simulink model "afe_abc_inv_psm_n"  (R2025b)
settings: Solver=ode1  StartTime=0.0  StopTime=simlength  FixedStep=tc  MaxStep=tc
values from neighbouring files (symbols this model uses):
  Adrso = eye(2) + Arso*ts_afe    [init_model.m]
  afe_pwm_phase_shift_mod1 = 0    [init_model.m]
  afe_pwm_phase_shift_mod2 = 0    [init_model.m]
  Aresd = eye(2) + Ares*ts_afe    [init_model.m]
  Bresd = Bres*ts_afe    [init_model.m]
  Cresd = Cres    [init_model.m]
  Crso = [1 0]    [init_model.m]
  CTRPIFF_CLIP_RELEASE = 0.001    [init_model.m]
  deepNEGeta = 0.5    [init_model.m]
  deepNEGxi = 0    [init_model.m]
  deepPOSxi = 0.5    [init_model.m]
  emf_fb_p = 0.2    [init_model.m]
  emf_fb_p_ccaller_1 = emf_fb_p    (= 0.2)    [init_model.m]
  emf_fb_p_ccaller_2 = emf_fb_p    (= 0.2)    [init_model.m]
  emf_p = emf_fb_p*4/10    (= 0.08)    [init_model.m]
  emf_p_ccaller_1 = emf_fb_p_ccaller_1*4/10    (= 0.08)    [init_model.m]
  emf_p_ccaller_2 = emf_fb_p_ccaller_2*4/10    (= 0.08)    [init_model.m]
  g0_161Hz = fcut_161Hz_flt * ts_afe * 2*pi    (= 0.126449104307)    [init_model.m]
  g0_1Hz = fcut_1Hz_flt * ts_afe * 2*pi    (= 0.000785398163397)    [init_model.m]
  g0_500Hz = fcut_500Hz_flt * ts_afe * 2*pi    (= 0.392699081699)    [init_model.m]
  g1_161Hz = 1 - g0_161Hz    (= 0.873550895693)    [init_model.m]
  g1_1Hz = 1 - g0_1Hz    (= 0.999214601837)    [init_model.m]
  g1_500Hz = 1 - g0_500Hz    (= 0.607300918301)    [init_model.m]
  i_grid_neg_eta_lim = 0.5    [init_model.m]
  i_grid_neg_eta_red_lim = 0.1    [init_model.m]
  i_grid_neg_xi_lim = 0.5    [init_model.m]
  i_grid_neg_xi_red_lim = 0.1    [init_model.m]
  i_grid_pos_eta_lim = 1    [init_model.m]
  i_grid_pos_eta_red_lim = 0.1    [init_model.m]
  id_lim = 0.35    [init_model.m]
  ieta_neg_ref_lim = 0.5    [init_model.m]
  ieta_pos_ref_lim = 1.0    (= 1)    [init_model.m]
  Igrid_phase_normalization_factor = 250e3/Vphase2/3/0.9*sqrt(2)    [init_model.m]
  inv_pwm_phase_shift_mod1 = 0    [init_model.m]
  iq_lim = 1.4    [init_model.m]
  ixi_pos_ref_lim = 1.6    [init_model.m]
  k_frt_ref = 2    [init_model.m]
  kg = Kobs(1)    [init_model.m]
  ki_afe = 45    [init_model.m]
  ki_align = 0.1    [init_model.m]
  ki_i = 18    [init_model.m]
  ki_rc_neg_grid = ki_rc_grid    (= 35)    [init_model.m]
  ki_rc_pos_grid = ki_rc_grid    (= 35)    [init_model.m]
  ki_vs = 35    [init_model.m]
  ki_w = 18    [init_model.m]
  kp_afe = 0.6    [init_model.m]
  kp_align = 0.6    [init_model.m]
  kp_i = 0.25    [init_model.m]
  kp_rc_neg_grid = kp_rc_grid    (= 0.35)    [init_model.m]
  kp_rc_pos_grid = kp_rc_grid    (= 0.35)    [init_model.m]
  kp_vs = 0.85    [init_model.m]
  kp_w = 2.5    [init_model.m]
  kw = Kobs(2)    [init_model.m]
  l1 = Kd(2)    [init_model.m]
  l2 = Kd(1)    [init_model.m]
  Ldrso = acker(Adrso',Crso',polesdrso)'    [init_model.m]
  lim_down_align = -0.2    [init_model.m]
  lim_up_align = 0.2    [init_model.m]
  mavarage_filter_frequency_base_order = 2    [init_model.m]
  motorc_m_scale = 2/3*Vdc_bez/ubez    [init_model.m]
  n1 = rms_perios/f_grid/ts_afe    [init_model.m]
  n10 = rms_perios/f_grid/ts_afe    [init_model.m]
  number_of_modules = 2    [init_model.m]
  omega_m_sim = omega_m_bez    [init_model.m]
  pll_i1 = 80    [init_model.m]
  pll_i1_ddsrt = pll_i1/2    (= 40)    [init_model.m]
  pll_p = 1    [init_model.m]
  pll_p_ddsrt = pll_p/2    (= 0.5)    [init_model.m]
  pll_p_frt = 0.2    [init_model.m]
  settle_time = 0.15    [init_model.m]
  simlength = 2    [init_model.m]
  start_time_LVRT = 2.0    (= 2)    [init_model.m]
  tc = ts_afe/200    (= 6.25e-07)    [init_model.m]
  time_aux_power_supply_fault = 1e3    (= 1000)    [init_model.m]
  time_gain_afe_module_1 = 1.0    (= 1)    [init_model.m]
  time_gain_afe_module_2 = 1.0    (= 1)    [init_model.m]
  time_gain_inv_module_1 = 1.0    (= 1)    [init_model.m]
  time_gain_inv_module_2 = 1.0    (= 1)    [init_model.m]
  time_phase_fault = 1e3    (= 1000)    [init_model.m]
  time_start_motor_control = 0.035    [init_model.m]
  transmission_delay = 125e-6*2    (= 0.00025)    [init_model.m]
  ts_afe = 1/fPWM_AFE/2    (= 0.000125)    [init_model.m]
  ts_inv = 1/fPWM_INV/2    (= 0.000125)    [init_model.m]
  Vdc_norm_ref = Vdc_ref/Vdc_nom    [init_model.m]
  Vdc_ref = 1070    [init_model.m]
  Vgrid_phase_normalization_factor = Vphase2*sqrt(2)    [init_model.m]
undefined symbols (not defined in the file or in its folder): Amplitude_U, Amplitude_V, Amplitude_W, end_time_LVRT, ibez, La, Lb, Ld_norm, Lq_norm, Ls_norm, magnitude, omega_bez, omega_grid_emulator_nom, omega_grid_nom, omega_m_bez, Phase_shift, psi_bez, psi_m, psi_m_norm, rpm_base, rpm_bez, Rs, Rs_norm, t_ramp, tau_bez, torque_base, ubez, ugrid_factor, V_phase_normalization_factor, Vdc_bez, Vemu_ref_norm, vn_eta_pu, vn_xi_pu, vp_xi_pu
libraries: fl_lib x215, nesl_utility x107, moving_average_filter x20, cstblocks x20, moving_average_filter_cc x16, simulink x6, threephase_inductor_lib x4, three_phase_pwm_modulator x4, single_phase_transformer_lib x3, power_meter_iec x1, flexshaft_lib x1, psm x1
(part 6 of 15)

== system afe_abc_inv_psm_n/afe_abc_inv_psm_mod1/AFE_control/afe_control/udc_ctrl ==
  udc_pu : Inport
  udc_pu_ref : Inport  Port=2
  1/Ti : Gain  Gain=kp_vs  SaturateOnIntegerOverflow=on  OutDataTypeStr=Inherit: Same as input  ParamDataTypeStr=Inherit: Same as input
  Constant : Constant  Value=0
  Gain : Gain  Gain=-1
  Saturation : Saturate  UpperLimit=ixi_pos_ref_lim  LowerLimit=-ixi_pos_ref_lim
  Sum1 : Sum  Inputs=+++  SaturateOnIntegerOverflow=on
  Sum2 : Sum  Inputs=-+  SaturateOnIntegerOverflow=on
  Sum3 : Sum  Inputs=-+  SaturateOnIntegerOverflow=on
  Switch : Switch  Criteria=u2 > Threshold  SaturateOnIntegerOverflow=off  InputSameDT=off
  To Workspace1 : ToWorkspace  VariableName=udc_pu_sim_mod1  SampleTime=-1
      settings: MaxDataPoints=Ns_afe
  To Workspace3 : ToWorkspace  VariableName=udc_pu_ref_sim_mod1  SampleTime=-1
      settings: MaxDataPoints=Ns_afe
  Unit Delay4 : UnitDelay  SampleTime=-1  HasFrameUpgradeWarning=on
  kp : Gain  Gain=ki_vs*ts_afe  SaturateOnIntegerOverflow=on  OutDataTypeStr=Inherit: Same as input  ParamDataTypeStr=Inherit: Same as input
  udc_tracking : Scope  NumInputPorts=2
      settings: ActiveDisplayYMinimum=-0.14752197265624997  ActiveDisplayYMaximum=1.32769775390625  DataLoggingVariableName=ScopeData8
  i_xi_ref : Outport
  wires:
  1/Ti/1 -> Sum1/1, Sum3/1
  kp/1 -> Sum1/2
  Sum3/1 -> Unit Delay4/1
  Unit Delay4/1 -> Sum1/3
  udc_pu_ref/1 -> To Workspace3/1, udc_tracking/1, Sum2/2  "udc_pu_ref"
  udc_pu/1 -> To Workspace1/1, udc_tracking/2, Sum2/1  "udc_pu"
  Sum2/1 -> kp/1, 1/Ti/1
  Sum1/1 -> Saturation/1
  Saturation/1 -> Gain/1, Sum3/2
  [pwr_lim_enable_mod1] -> Switch/2
  Gain/1 -> Switch/3
  Switch/1 -> i_xi_ref/1
  Constant/1 -> Switch/1

== system afe_abc_inv_psm_n/afe_abc_inv_psm_mod1/AFE_control/afe_control/ug afe quantizzation and one step delay ==
  ug_abc_pu : Inport
  Demux : Demux  Outputs=3
  Mux : Mux  Inputs=3
  ug afe quantizzation and one step delay : Subsystem
  ugd_abc_pu : Outport
  wires:
  ug afe quantizzation and one step delay/2(ugd_v_pu) -> Mux/2
  Demux/2 -> ug afe quantizzation and one step delay/2(ug_v_pu)
  Demux/3 -> ug afe quantizzation and one step delay/3(ug_w_pu)
  ug afe quantizzation and one step delay/1(ugd_u_pu) -> Mux/1
  Demux/1 -> ug afe quantizzation and one step delay/1(ug_u_pu)
  ug_abc_pu/1 -> Demux/1
  ug afe quantizzation and one step delay/3(ugd_w_pu) -> Mux/3
  Mux/1 -> ugd_abc_pu/1

== system afe_abc_inv_psm_n/afe_abc_inv_psm_mod1/INV_control/inverter_control/Speed control ==
  rotor speed : Inport
  rotor speed ref : Inport  Port=2
  1/Ti : Gain  Gain=kp_w  SaturateOnIntegerOverflow=on  OutDataTypeStr=Inherit: Same as input  ParamDataTypeStr=Inherit: Same as input
  Saturation : Saturate  UpperLimit=iq_lim  LowerLimit=-iq_lim
  Sum1 : Sum  Inputs=+++  SaturateOnIntegerOverflow=on
  Sum2 : Sum  Inputs=-+  SaturateOnIntegerOverflow=on
  Sum3 : Sum  Inputs=-+  SaturateOnIntegerOverflow=on
  Unit Delay4 : UnitDelay  SampleTime=-1  HasFrameUpgradeWarning=on
  kp : Gain  Gain=ki_w*ts_inv  SaturateOnIntegerOverflow=on  OutDataTypeStr=Inherit: Same as input  ParamDataTypeStr=Inherit: Same as input
  torque_ref : Outport
  wires:
  1/Ti/1 -> Sum1/1, Sum3/1
  kp/1 -> Sum1/2
  Sum3/1 -> Unit Delay4/1
  Unit Delay4/1 -> Sum1/3
  rotor speed ref/1 -> Sum2/2
  rotor speed/1 -> Sum2/1
  Sum2/1 -> kp/1, 1/Ti/1
  Sum1/1 -> Saturation/1
  Saturation/1 -> Sum3/2, torque_ref/1

== system afe_abc_inv_psm_n/afe_abc_inv_psm_mod1/INV_control/inverter_control/current_ctrl ==
  torque_ref : Inport
  Bus Creator1 : BusCreator  Inputs=2
  bemf_observer : Subsystem
  current_ctrl : Subsystem
  current_transformation : Subsystem
  uab : Outport  VectorParamsAs1DForOutWhenUnconnected=off
  wires:
  [ubeta_pu_mod1] -> Bus Creator1/2  "ub"
  [ualpha_pu_mod1] -> Bus Creator1/1  "ua"
  Bus Creator1/1 -> uab/1
  torque_ref/1 -> current_ctrl/1(iq_ref)  "torque_ref"
  [ibeta_pu_mod1] -> bemf_observer/2(ibeta_pu)
  [ialpha_pu_mod1] -> bemf_observer/1(ialpha_pu)
  [ualpha_pu_mod1] -> bemf_observer/3(ualpha_pu)
  [ubeta_pu_mod1] -> bemf_observer/4(ubeta_pu)
  [udcd_pu_inv_mod1] -> current_ctrl/2(udc_pu), bemf_observer/5(udc_pu)

== system afe_abc_inv_psm_n/afe_abc_inv_psm_mod1/INV_control/inverter_control/encoder-sensorless-switch ==
  theta_elec_psm : Inport
  Variant Source1 : VariantSource  VariantControls={use_psm_encoder == 1, use_psm_encoder == 0}
  Variant Source2 : VariantSource  VariantControls={use_psm_encoder == 1, use_psm_encoder == 0}
  double_integrator_observer : Subsystem
  omega_pu_psm/hat1 : Scope  NumInputPorts=2
      settings: ActiveDisplayYMinimum=-0.11085278602064572  ActiveDisplayYMaximum=0.99767500251710517  DataLoggingVariableName=ScopeData13
  theta_elec_psm/hat : Scope  NumInputPorts=2
      settings: ActiveDisplayYMinimum=-3.9234912991523743  ActiveDisplayYMaximum=3.9263074994087219  DataLoggingVariableName=ScopeData12
  tag scope: motor_phase_ctrl_mod1=global, motor_speed_pu_ctrl_mod1=global
  wires:
  double_integrator_observer/1(omega_pu_psm_hat) -> omega_pu_psm/hat1/2, Variant Source1/1  "omega_pu_psm_hat"
  [theta_hat_mod1] -> Variant Source2/2  "theta_hat_mod1"
  theta_elec_psm/1 -> theta_elec_psm/hat/2, double_integrator_observer/1(theta_psm)  "theta_elec_psm"
  double_integrator_observer/2(theta_psm_hat) -> Variant Source2/1  "theta_psm_hat"
  [omega_hat_pu_mod1] -> Variant Source1/2  "omega_hat_pu_mod1"
  Variant Source1/1 -> [motor_speed_pu_ctrl_mod1]
  Variant Source2/1 -> [motor_phase_ctrl_mod1]
  [theta_hat_mod1] -> theta_elec_psm/hat/1  "theta_hat_mod1"
  [omega_hat_pu_mod1] -> omega_pu_psm/hat1/1  "omega_hat_pu_mod1"

== system afe_abc_inv_psm_n/afe_abc_inv_psm_mod1/INV_control/inverter_control/is inv quantizzation and one step delay ==
  is_abc_pu : Inport
  Demux : Demux  Outputs=3
  Mux : Mux  Inputs=3
  is inv quantizzation and one step delay : Subsystem
  isd_abc_pu : Outport
  wires:
  is inv quantizzation and one step delay/2(isd_v_pu) -> Mux/2
  is_abc_pu/1 -> Demux/1
  is inv quantizzation and one step delay/3(isd_w_pu) -> Mux/3
  is inv quantizzation and one step delay/1(isd_u_pu) -> Mux/1
  Demux/1 -> is inv quantizzation and one step delay/1(is_u_pu)
  Mux/1 -> isd_abc_pu/1
  Demux/3 -> is inv quantizzation and one step delay/3(is_w_pu)
  Demux/2 -> is inv quantizzation and one step delay/2(is_v_pu)

== system afe_abc_inv_psm_n/afe_abc_inv_psm_mod1/INV_control/inverter_control/measurements ==
  Gain : Gain  Gain=psi_bez
  Gain1 : Gain  Gain=psi_bez
  To Workspace10 : ToWorkspace  VariableName=id_pu_sim_mod1  SampleTime=-1
      settings: MaxDataPoints=Ns_inv
  To Workspace11 : ToWorkspace  VariableName=iq_pu_sim_mod1  SampleTime=-1
      settings: MaxDataPoints=Ns_inv
  To Workspace12 : ToWorkspace  VariableName=uq_pu_sim_mod1  SampleTime=-1
      settings: MaxDataPoints=Ns_inv
  To Workspace13 : ToWorkspace  VariableName=iq_pu_ref_sim_mod1  SampleTime=-1
      settings: MaxDataPoints=Ns_inv
  To Workspace14 : ToWorkspace  VariableName=id_pu_ref_sim_mod1  SampleTime=-1
      settings: MaxDataPoints=Ns_inv
  To Workspace15 : ToWorkspace  VariableName=u_mot_pu_sim_mod1  SampleTime=-1
      settings: MaxDataPoints=Ns_inv
  To Workspace2 : ToWorkspace  VariableName=ualpha_pu_sim_mod1  SampleTime=-1
      settings: MaxDataPoints=Ns_inv
  To Workspace3 : ToWorkspace  VariableName=ubeta_pu_sim_mod1  SampleTime=-1
      settings: MaxDataPoints=Ns_inv
  To Workspace4 : ToWorkspace  VariableName=psi_pu_alpha_hat_sim_mod1  SampleTime=-1
      settings: MaxDataPoints=Ns_inv
  To Workspace5 : ToWorkspace  VariableName=psi_pu_beta_hat_sim_mod1  SampleTime=-1
      settings: MaxDataPoints=Ns_inv
  To Workspace6 : ToWorkspace  VariableName=psi_r_alpha_hat_sim_mod1  SampleTime=-1
      settings: MaxDataPoints=Ns_inv
  To Workspace7 : ToWorkspace  VariableName=ud_pu_sim_mod1  SampleTime=-1
      settings: MaxDataPoints=Ns_inv
  To Workspace8 : ToWorkspace  VariableName=psi_r_beta_hat_sim_mod1  SampleTime=-1
      settings: MaxDataPoints=Ns_inv
  wires:
  [psi_r_alpha_pu_hat_mod1] -> Gain/1
  [ualpha_pu_mod1] -> To Workspace2/1  "ualpha_pu_mod1"
  Gain/1 -> To Workspace6/1  "psi_r_alpha_hat"
  [psi_r_alpha_pu_hat_mod1] -> To Workspace4/1  "phi_alpha_pu_hat"
  [ubeta_pu_mod1] -> To Workspace3/1  "ubeta_pu_mod1"
  [psi_r_beta_pu_hat_mod1] -> To Workspace5/1  "phi_beta_pu_hat"
  Gain1/1 -> To Workspace8/1  "psi_r_beta_hat"
  [psi_r_beta_pu_hat_mod1] -> Gain1/1
  [u_mot_pu_mod1] -> To Workspace15/1  "u_mot_pu_mod1"
  [iq_pu_ref_mod1] -> To Workspace13/1  "iq_pu_ref_mod1"
  [ud_pu_mod1] -> To Workspace7/1  "ud_pu_mod1"
  [uq_pu_mod1] -> To Workspace12/1  "uq_pu_mod1"
  [iq_pu_mod1] -> To Workspace11/1  "iq_pu_mod1"
  [id_pu_mod1] -> To Workspace10/1  "id_pu_mod1"
  [id_pu_ref_mod1] -> To Workspace14/1  "id_pu_ref_mod1"

== system afe_abc_inv_psm_n/afe_abc_inv_psm_mod1/INV_control/inverter_control/omega_pu ==
  Abs : Abs  SaturateOnIntegerOverflow=off
  flt : Subsystem
  abs(omega_pu) : Outport
  omega_pu : Outport  Port=2
  wires:
  Abs/1 -> flt/1(input)
  [motor_speed_pu_ctrl_mod1] -> Abs/1, omega_pu/1
  flt/1(output) -> abs(omega_pu)/1

== system afe_abc_inv_psm_n/afe_abc_inv_psm_mod1/INV_control/inverter_control/phase_compensation_1 ==
  local_time : Inport
  master_time : Inport  Port=2
  alignment_ctrl : Subsystem
  y : Outport
  wires:
  local_time/1 -> alignment_ctrl/1(local_time)
  master_time/1 -> alignment_ctrl/2(master_time)
  alignment_ctrl/1(dp) -> y/1

== system afe_abc_inv_psm_n/afe_abc_inv_psm_mod1/INV_control/inverter_control/space_vector ==
  uab_out : Inport
  Bus Creator : BusCreator  Inputs=3
  Bus Selector : BusSelector  OutputSignals=da,db,dc
  Bus Selector1 : BusSelector  OutputSignals=ua,ub
  C Caller : CCaller  FunctionName=sv_pwm_process_simulink  PortSpecificationStruct="%)30     .    V @   8    (     @         %    \"     4    !     0         %  0 \"0    $    _    07)G3F%M90  4&]R=$YA;64 4V-O<&4     26YD97@     5'EP90      4VEZ90      27-';&]B86P   X    P    !@    @    $          4    (     0    ,    !         !   P!O=70 #@   #     &    \"     0         !0    @    !     P    $         $  # &]U=  .    .     8    (    !          %    \"     $    &     0         0   ...(+2669 chars)"
  Constant : Constant  Value=ts_inv
  Constant1 : Constant
  Data Type Conversion1 : DataTypeConversion  OutDataTypeStr=double  SaturateOnIntegerOverflow=off  RndMeth=Floor
  Data Type Conversion15 : DataTypeConversion  OutDataTypeStr=single  SaturateOnIntegerOverflow=off  RndMeth=Floor
  Data Type Conversion16 : DataTypeConversion  OutDataTypeStr=single  SaturateOnIntegerOverflow=off  RndMeth=Floor
  Data Type Conversion17 : DataTypeConversion  OutDataTypeStr=uint32  SaturateOnIntegerOverflow=off  RndMeth=Floor
  Data Type Conversion18 : DataTypeConversion  OutDataTypeStr=single  SaturateOnIntegerOverflow=off  RndMeth=Floor
  Data Type Conversion2 : DataTypeConversion  OutDataTypeStr=double  SaturateOnIntegerOverflow=off  RndMeth=Floor
  Data Type Conversion3 : DataTypeConversion  OutDataTypeStr=double  SaturateOnIntegerOverflow=off  RndMeth=Floor
  Gain1 : Gain  Gain=sqrt(3)/2
  Gain2 : Gain  Gain=sqrt(3)/2
  duvw : Outport
  wires:
  Data Type Conversion15/1 -> C Caller/2
  Bus Selector/2 -> Data Type Conversion2/1  "<db>"
  Data Type Conversion16/1 -> C Caller/3
  Data Type Conversion18/1 -> C Caller/1
  C Caller/1 -> Bus Selector/1
  Bus Creator/1 -> duvw/1
  Data Type Conversion17/1 -> C Caller/4
  Data Type Conversion1/1 -> Bus Creator/1  "du(k)"
  Bus Selector1/2 -> Gain2/1  "<ub>"
  Bus Selector/3 -> Data Type Conversion3/1  "<dc>"
  Bus Selector1/1 -> Gain1/1  "<ua>"
  Data Type Conversion2/1 -> Bus Creator/2  "dv(k)"
  Gain2/1 -> Data Type Conversion15/1
  Bus Selector/1 -> Data Type Conversion1/1  "<da>"
  Gain1/1 -> Data Type Conversion18/1
  Data Type Conversion3/1 -> Bus Creator/3  "dw(k)"
  Constant/1 -> Data Type Conversion16/1
  uab_out/1 -> Bus Selector1/1
  Constant1/1 -> Data Type Conversion17/1

== system afe_abc_inv_psm_n/afe_abc_inv_psm_mod1/INV_control/inverter_control/speed_reference_generator ==
  Step : Step  Time=time_start_motor_control  After=omega_m_sim/omega_m_bez
  Step1 : Step  Commented=on  Time=simlength/2  After=-2*omega_m_sim/omega_m_bez
  Sum : Sum  Inputs=|++
  flt : Subsystem
  omega_ref_pu : Outport
  tag scope: omega_ref_pu_mod1=global
  wires:
  Step/1 -> Sum/1
  Step1/1 -> Sum/2
  Sum/1 -> flt/1(input)
  flt/1(output) -> [omega_ref_pu_mod1], omega_ref_pu/1

== system afe_abc_inv_psm_n/afe_abc_inv_psm_mod1/INV_control/inverter_control/torque_reference ==
  rotor speed : Inport
  1-D Lookup Table : Lookup_n-D  NumberOfTableDimensions=1  BreakpointsForDimension1=rpm_base  Table=torque_base  InternalRulePriority=Speed  RndMeth=Simplest
  Gain : Gain  Gain=-1.25
  Gain1 : Gain  Gain=1/tau_bez
  Gain2 : Gain  Gain=rpm_bez
  Saturation : Saturate  UpperLimit=0  LowerLimit=-inf
  torque_ref : Outport
  wires:
  rotor speed/1 -> Gain2/1
  Gain/1 -> Saturation/1
  Saturation/1 -> torque_ref/1
  Gain1/1 -> Gain/1
  1-D Lookup Table/1 -> Gain1/1
  Gain2/1 -> 1-D Lookup Table/1

== system afe_abc_inv_psm_n/afe_abc_inv_psm_mod1/INV_control/inverter_control/udc_acquisition ==
  udc_pu : Inport
  Quantizer : Quantizer  QuantizationInterval=adc_quantization
  Unit Delay : UnitDelay  SampleTime=-1  HasFrameUpgradeWarning=on
  udcd_pu : Outport
  wires:
  Quantizer/1 -> Unit Delay/1
  udc_pu/1 -> Quantizer/1
  Unit Delay/1 -> udcd_pu/1

== system afe_abc_inv_psm_n/afe_abc_inv_psm_mod1/afe/dclink_measure/R_derating ==
  Step : Step  After=107.4e3/2  SampleTime=0
  Step1 : Step  Time=1.1  After=-107.4e3/2  SampleTime=0
  Sum : Sum  Inputs=|++
  DR : Outport
  wires:
  Step1/1 -> Sum/2
  Step/1 -> Sum/1
  Sum/1 -> DR/1

== system afe_abc_inv_psm_n/afe_abc_inv_psm_mod1/afe/sv_pwm/modulator1 ==
  u : Inport
  v : Inport  Port=2
  w : Inport  Port=3
  phase : Inport  Port=4
  Bus Creator : BusCreator  Inputs=3
  Three phase two level PWM generator with global TRGO : three_phase_pwm_modulator/Three phase two level PWM generator with global TRGO  f=fPWM_AFE  m_up=0.98  m_low=0.02  dead_time=dead_time_AFE  pos_cmd_gate=15  neg_cmd_gate=-10  polarity=1  tc=tc  double_sampling=1
      link override gate commands/Bus Selector: OutputSignals=du(t)
      link override gate commands/Bus Selector1: OutputSignals=dv(t)
      link override gate commands/Bus Selector2: OutputSignals=dw(t)
  gate_cmds : Outport
  tag scope: TRGO_afe_module_1=global
  wires:
  [time_afe_module_1] -> Three phase two level PWM generator with global TRGO/1
  Bus Creator/1 -> Three phase two level PWM generator with global TRGO/3
  Three phase two level PWM generator with global TRGO/1 -> [TRGO_afe_module_1]
  u/1 -> Bus Creator/1
  v/1 -> Bus Creator/2
  w/1 -> Bus Creator/3
  phase/1 -> Three phase two level PWM generator with global TRGO/2
  Three phase two level PWM generator with global TRGO/2 -> gate_cmds/1

== system afe_abc_inv_psm_n/afe_abc_inv_psm_mod1/inverter/inverter/sv_pwm ==
  duties_uvw : Inport
  Bus Selector2 : BusSelector  OutputSignals=du(k),dv(k),dw(k)
  Constant1 : Constant  Value=inv_pwm_phase_shift_mod1
  modulator1 : Subsystem
  td2tc_1 : TransferFcn  Denominator=[tc 1]
  td2tc_2 : TransferFcn  Denominator=[tc 1]
  td2tc_3 : TransferFcn  Denominator=[tc 1]
  gate_cmds : Outport
  wires:
  modulator1/1(gate_cmds) -> gate_cmds/1
  Constant1/1 -> modulator1/4(phase)
  Bus Selector2/1 -> td2tc_1/1  "<du(k)>"
  Bus Selector2/2 -> td2tc_2/1  "<dv(k)>"
  Bus Selector2/3 -> td2tc_3/1  "<dw(k)>"
  duties_uvw/1 -> Bus Selector2/1
  td2tc_1/1 -> modulator1/1(u)  "du(t)"
  td2tc_3/1 -> modulator1/3(w)  "dw(t)"
  td2tc_2/1 -> modulator1/2(v)  "dv(t)"

== system afe_abc_inv_psm_n/afe_abc_inv_psm_mod1/inverter/inverter/switch_1 ==
  Diode : fl_lib/Electrical/Electrical Elements/Diode  Vf=Vgamma V  Ron=Ron Ohm  Goff=1e-8 1/Ohm  i_specify=off  i_priority=None  i=0 A  i_nominal_specify=off  i_nominal_value=1  i_nominal_unit=A  v_specify=off  v_priority=None  v=0 V  v_nominal_specify=off  v_nominal_value=1  v_nominal_unit=V
  Switch : fl_lib/Electrical/Electrical Elements/Switch  R_closed=Ron Ohm  G_open=1e-8 1/Ohm  Threshold=7.5  i_specify=off  i_priority=None  i=0 A  i_nominal_specify=off  i_nominal_value=1  i_nominal_unit=A  v_specify=off  v_priority=None  v=0 V  v_nominal_specify=off  v_nominal_value=1  v_nominal_unit=V
  snubber : fl_lib/Electrical/Electrical Elements/Capacitor  c=Csnubber F  r=Rsnubber Ohm  g=0 1/Ohm  i_specify=off  i_priority=None  i=0 A  i_nominal_specify=off  i_nominal_value=1  i_nominal_unit=A  v_specify=off  v_priority=None  v=0 V  v_nominal_specify=off  v_nominal_value=1  v_nominal_unit=V  vc_specify=off  vc_priority=High  vc=0 V  vc_nominal_specify=off  vc_nominal_value=1  vc_nominal_unit=V
  G : PMIOPort  Side=Left
  C : PMIOPort  Port=2  Side=Left
  E : PMIOPort  Port=3  Side=Right
  connections:
  Switch/RConn2 -- C/RConn1 -- snubber/LConn1 -- Diode/RConn1
  Switch/RConn1 -- G/RConn1
  Switch/LConn1 -- E/RConn1 -- snubber/RConn1 -- Diode/LConn1

== system afe_abc_inv_psm_n/afe_abc_inv_psm_mod1/inverter/inverter/switch_2 ==
  Diode : fl_lib/Electrical/Electrical Elements/Diode  Vf=Vgamma V  Ron=Ron Ohm  Goff=1e-8 1/Ohm  i_specify=off  i_priority=None  i=0 A  i_nominal_specify=off  i_nominal_value=1  i_nominal_unit=A  v_specify=off  v_priority=None  v=0 V  v_nominal_specify=off  v_nominal_value=1  v_nominal_unit=V
  Switch : fl_lib/Electrical/Electrical Elements/Switch  R_closed=Ron Ohm  G_open=1e-8 1/Ohm  Threshold=7.5  i_specify=off  i_priority=None  i=0 A  i_nominal_specify=off  i_nominal_value=1  i_nominal_unit=A  v_specify=off  v_priority=None  v=0 V  v_nominal_specify=off  v_nominal_value=1  v_nominal_unit=V
  snubber : fl_lib/Electrical/Electrical Elements/Capacitor  c=Csnubber F  r=Rsnubber Ohm  g=0 1/Ohm  i_specify=off  i_priority=None  i=0 A  i_nominal_specify=off  i_nominal_value=1  i_nominal_unit=A  v_specify=off  v_priority=None  v=0 V  v_nominal_specify=off  v_nominal_value=1  v_nominal_unit=V  vc_specify=off  vc_priority=High  vc=0 V  vc_nominal_specify=off  vc_nominal_value=1  vc_nominal_unit=V
  G : PMIOPort  Side=Left
  C : PMIOPort  Port=2  Side=Left
  E : PMIOPort  Port=3  Side=Right
  connections:
  snubber/RConn1 -- E/RConn1 -- Switch/LConn1 -- Diode/LConn1
  Switch/RConn1 -- G/RConn1
  snubber/LConn1 -- Diode/RConn1 -- C/RConn1 -- Switch/RConn2

== system afe_abc_inv_psm_n/afe_abc_inv_psm_mod1/inverter/inverter/switch_3 ==
  Diode : fl_lib/Electrical/Electrical Elements/Diode  Vf=Vgamma V  Ron=Ron Ohm  Goff=1e-8 1/Ohm  i_specify=off  i_priority=None  i=0 A  i_nominal_specify=off  i_nominal_value=1  i_nominal_unit=A  v_specify=off  v_priority=None  v=0 V  v_nominal_specify=off  v_nominal_value=1  v_nominal_unit=V
  Switch : fl_lib/Electrical/Electrical Elements/Switch  R_closed=Ron Ohm  G_open=1e-8 1/Ohm  Threshold=7.5  i_specify=off  i_priority=None  i=0 A  i_nominal_specify=off  i_nominal_value=1  i_nominal_unit=A  v_specify=off  v_priority=None  v=0 V  v_nominal_specify=off  v_nominal_value=1  v_nominal_unit=V
  snubber : fl_lib/Electrical/Electrical Elements/Capacitor  c=Csnubber F  r=Rsnubber Ohm  g=0 1/Ohm  i_specify=off  i_priority=None  i=0 A  i_nominal_specify=off  i_nominal_value=1  i_nominal_unit=A  v_specify=off  v_priority=None  v=0 V  v_nominal_specify=off  v_nominal_value=1  v_nominal_unit=V  vc_specify=off  vc_priority=High  vc=0 V  vc_nominal_specify=off  vc_nominal_value=1  vc_nominal_unit=V
  G : PMIOPort  Side=Left
  C : PMIOPort  Port=2  Side=Left
  E : PMIOPort  Port=3  Side=Right
  connections:
  Switch/RConn2 -- C/RConn1 -- Diode/RConn1 -- snubber/LConn1
  Switch/RConn1 -- G/RConn1
  Diode/LConn1 -- Switch/LConn1 -- E/RConn1 -- snubber/RConn1

== system afe_abc_inv_psm_n/afe_abc_inv_psm_mod1/inverter/inverter/switch_4 ==
  Diode : fl_lib/Electrical/Electrical Elements/Diode  Vf=Vgamma V  Ron=Ron Ohm  Goff=1e-8 1/Ohm  i_specify=off  i_priority=None  i=0 A  i_nominal_specify=off  i_nominal_value=1  i_nominal_unit=A  v_specify=off  v_priority=None  v=0 V  v_nominal_specify=off  v_nominal_value=1  v_nominal_unit=V
  Switch : fl_lib/Electrical/Electrical Elements/Switch  R_closed=Ron Ohm  G_open=1e-8 1/Ohm  Threshold=7.5  i_specify=off  i_priority=None  i=0 A  i_nominal_specify=off  i_nominal_value=1  i_nominal_unit=A  v_specify=off  v_priority=None  v=0 V  v_nominal_specify=off  v_nominal_value=1  v_nominal_unit=V
  snubber : fl_lib/Electrical/Electrical Elements/Capacitor  c=Csnubber F  r=Rsnubber Ohm  g=0 1/Ohm  i_specify=off  i_priority=None  i=0 A  i_nominal_specify=off  i_nominal_value=1  i_nominal_unit=A  v_specify=off  v_priority=None  v=0 V  v_nominal_specify=off  v_nominal_value=1  v_nominal_unit=V  vc_specify=off  vc_priority=High  vc=0 V  vc_nominal_specify=off  vc_nominal_value=1  vc_nominal_unit=V
  G : PMIOPort  Side=Left
  C : PMIOPort  Port=2  Side=Left
  E : PMIOPort  Port=3  Side=Right
  connections:
  snubber/RConn1 -- E/RConn1 -- Switch/LConn1 -- Diode/LConn1
  Switch/RConn1 -- G/RConn1
  snubber/LConn1 -- Diode/RConn1 -- C/RConn1 -- Switch/RConn2

== system afe_abc_inv_psm_n/afe_abc_inv_psm_mod1/inverter/inverter/switch_5 ==
  Diode : fl_lib/Electrical/Electrical Elements/Diode  Vf=Vgamma V  Ron=Ron Ohm  Goff=1e-8 1/Ohm  i_specify=off  i_priority=None  i=0 A  i_nominal_specify=off  i_nominal_value=1  i_nominal_unit=A  v_specify=off  v_priority=None  v=0 V  v_nominal_specify=off  v_nominal_value=1  v_nominal_unit=V
  Switch : fl_lib/Electrical/Electrical Elements/Switch  R_closed=Ron Ohm  G_open=1e-8 1/Ohm  Threshold=7.5  i_specify=off  i_priority=None  i=0 A  i_nominal_specify=off  i_nominal_value=1  i_nominal_unit=A  v_specify=off  v_priority=None  v=0 V  v_nominal_specify=off  v_nominal_value=1  v_nominal_unit=V
  snubber : fl_lib/Electrical/Electrical Elements/Capacitor  c=Csnubber F  r=Rsnubber Ohm  g=0 1/Ohm  i_specify=off  i_priority=None  i=0 A  i_nominal_specify=off  i_nominal_value=1  i_nominal_unit=A  v_specify=off  v_priority=None  v=0 V  v_nominal_specify=off  v_nominal_value=1  v_nominal_unit=V  vc_specify=off  vc_priority=High  vc=0 V  vc_nominal_specify=off  vc_nominal_value=1  vc_nominal_unit=V
  G : PMIOPort  Side=Left
  C : PMIOPort  Port=2  Side=Left
  E : PMIOPort  Port=3  Side=Right
  connections:
  Switch/RConn2 -- C/RConn1 -- Diode/RConn1 -- snubber/LConn1
  Switch/RConn1 -- G/RConn1
  Diode/LConn1 -- Switch/LConn1 -- E/RConn1 -- snubber/RConn1

== system afe_abc_inv_psm_n/afe_abc_inv_psm_mod1/inverter/inverter/switch_6 ==
  Diode : fl_lib/Electrical/Electrical Elements/Diode  Vf=Vgamma V  Ron=Ron Ohm  Goff=1e-8 1/Ohm  i_specify=off  i_priority=None  i=0 A  i_nominal_specify=off  i_nominal_value=1  i_nominal_unit=A  v_specify=off  v_priority=None  v=0 V  v_nominal_specify=off  v_nominal_value=1  v_nominal_unit=V
  Switch : fl_lib/Electrical/Electrical Elements/Switch  R_closed=Ron Ohm  G_open=1e-8 1/Ohm  Threshold=7.5  i_specify=off  i_priority=None  i=0 A  i_nominal_specify=off  i_nominal_value=1  i_nominal_unit=A  v_specify=off  v_priority=None  v=0 V  v_nominal_specify=off  v_nominal_value=1  v_nominal_unit=V
  snubber : fl_lib/Electrical/Electrical Elements/Capacitor  c=Csnubber F  r=Rsnubber Ohm  g=0 1/Ohm  i_specify=off  i_priority=None  i=0 A  i_nominal_specify=off  i_nominal_value=1  i_nominal_unit=A  v_specify=off  v_priority=None  v=0 V  v_nominal_specify=off  v_nominal_value=1  v_nominal_unit=V  vc_specify=off  vc_priority=High  vc=0 V  vc_nominal_specify=off  vc_nominal_value=1  vc_nominal_unit=V
  G : PMIOPort  Side=Left
  C : PMIOPort  Port=2  Side=Left
  E : PMIOPort  Port=3  Side=Right
  connections:
  snubber/RConn1 -- E/RConn1 -- Switch/LConn1 -- Diode/LConn1
  Switch/RConn1 -- G/RConn1
  snubber/LConn1 -- Diode/RConn1 -- C/RConn1 -- Switch/RConn2

== system afe_abc_inv_psm_n/afe_abc_inv_psm_mod2/AFE_control/afe_control/FRT-VDE4110 ==
  FRT-Detection : Subsystem
  FRT-PosNegReactiveCurrentReferences : Subsystem
  frt_detection_output : Scope  NumInputPorts=3
      settings: ActiveDisplayYMinimum=-0.125  ActiveDisplayYMaximum=1.125
  tag scope: frt_active_mod2=global, pwr_lim_enable_mod2=global
  wires:
  FRT-Detection/2(frt_state) -> frt_detection_output/1  "frt_state"
  FRT-Detection/5(pwr_lim_enable) -> [pwr_lim_enable_mod2], frt_detection_output/3  "pwr_lim_enable"
  FRT-Detection/4(frt_active) -> [frt_active_mod2], frt_detection_output/2  "frt_active"
  [v_grid_pos_eta_avg_mod2] -> FRT-PosNegReactiveCurrentReferences/2(In2)
  [v_grid_neg_eta_avg_mod2] -> FRT-PosNegReactiveCurrentReferences/4(In4)
  [v_grid_neg_xi_avg_mod2] -> FRT-PosNegReactiveCurrentReferences/3(In3)
  [v_grid_pos_xi_avg_mod2] -> FRT-PosNegReactiveCurrentReferences/1(In1)

== system afe_abc_inv_psm_n/afe_abc_inv_psm_mod2/AFE_control/afe_control/current_ctrl ==
  i_xi_ref : Inport
  is_abc_pu : Inport  Port=2
  Demux : Demux  Outputs=3
  Inner Loop Current Control : Subsystem
  current_transformation : Subsystem
  xieta2abc : Subsystem
  uab_out : Outport
  wires:
  [i_stack_pos_eta_ref_mod2] -> xieta2abc/2(pos_eta)
  [i_stack_neg_xi_ref_mod2] -> xieta2abc/3(neg_xi)
  [i_stack_neg_eta_ref_mod2] -> xieta2abc/4(neg_eta)
  i_xi_ref/1 -> xieta2abc/1(pos_xi)  "i_xi_ref"
  Inner Loop Current Control/1(uab) -> uab_out/1
  [isd_abc_pu_mod2] -> Inner Loop Current Control/2(is_abc)
  xieta2abc/1(i_abc) -> Inner Loop Current Control/1(In1)
  [gamma_grid_pll_mod2] -> xieta2abc/5(gamma)
  is_abc_pu/1 -> Demux/1
  Demux/3 -> current_transformation/3(is_c_pu)  "is_c"
  Demux/2 -> current_transformation/2(is_b_pu)  "is_b"
  Demux/1 -> current_transformation/1(is_a_pu)  "is_a"

== system afe_abc_inv_psm_n/afe_abc_inv_psm_mod2/AFE_control/afe_control/data_to_worspace_module_1 ==
  Bus Selector : BusSelector  OutputSignals=i_grid_pos_eta_ref,i_grid_neg_eta_ref,i_grid_neg_xi_ref
  To Workspace1 : ToWorkspace  VariableName=i_grid_pos_eta_ref_sim_mod2  SampleTime=-1
      settings: MaxDataPoints=Ns_afe
  To Workspace11 : ToWorkspace  VariableName=i_grid_pos_xi_sim_mod2  SampleTime=-1
      settings: MaxDataPoints=Ns_afe
  To Workspace13 : ToWorkspace  VariableName=i_grid_pos_eta_sim_mod2  SampleTime=-1
      settings: MaxDataPoints=Ns_afe
  To Workspace14 : ToWorkspace  VariableName=i_grid_neg_xi_sim_mod2  SampleTime=-1
      settings: MaxDataPoints=Ns_afe
  To Workspace15 : ToWorkspace  VariableName=i_grid_neg_eta_sim_mod2  SampleTime=-1
      settings: MaxDataPoints=Ns_afe
  To Workspace16 : ToWorkspace  VariableName=u_grid_pos_xi_sim_mod2  SampleTime=-1
      settings: MaxDataPoints=Ns_afe
  To Workspace17 : ToWorkspace  VariableName=u_grid_pos_eta_sim_mod2  SampleTime=-1
      settings: MaxDataPoints=Ns_afe
  To Workspace18 : ToWorkspace  VariableName=u_grid_neg_xi_sim_mod2  SampleTime=-1
      settings: MaxDataPoints=Ns_afe
  To Workspace19 : ToWorkspace  VariableName=u_grid_neg_eta_sim_mod2  SampleTime=-1
      settings: MaxDataPoints=Ns_afe
  To Workspace2 : ToWorkspace  VariableName=i_grid_neg_xi_ref_sim_mod2  SampleTime=-1
      settings: MaxDataPoints=Ns_afe
  To Workspace3 : ToWorkspace  VariableName=i_grid_neg_eta_ref_sim_mod2  SampleTime=-1
      settings: MaxDataPoints=Ns_afe
  wires:
  Bus Selector/3 -> To Workspace2/1  "<i_grid_neg_xi_ref>"
  Bus Selector/2 -> To Workspace3/1  "<i_grid_neg_eta_ref>"
  Bus Selector/1 -> To Workspace1/1  "<i_grid_pos_eta_ref>"
  [i_grid_seq_ref_mod2] -> Bus Selector/1
  [v_grid_neg_xi_avg_mod2] -> To Workspace18/1
  [v_grid_pos_eta_avg_mod2] -> To Workspace17/1
  [v_grid_neg_eta_avg_mod2] -> To Workspace19/1
  [v_grid_pos_xi_avg_mod2] -> To Workspace16/1
  [i_grid_neg_eta_avg_mod2] -> To Workspace15/1
  [i_grid_neg_xi_avg_mod2] -> To Workspace14/1
  [i_grid_pos_xi_avg_mod2] -> To Workspace11/1
  [i_grid_pos_eta_avg_mod2] -> To Workspace13/1

== system afe_abc_inv_psm_n/afe_abc_inv_psm_mod2/AFE_control/afe_control/grid_current_sequences_and_reactive_pwr_ctrl ==
  ig_abc_pu : Inport
  current_sequence_avg : Subsystem
  grid_current_sampling_and_alpha_beta_transformation : Subsystem
  i_alphabeta2xieta : Subsystem
  sequences_current_control : Subsystem
  tag scope: i_grid_neg_eta_avg_mod2=global, i_grid_neg_xi_avg_mod2=global, i_grid_pos_eta_avg_mod2=global, i_grid_pos_xi_avg_mod2=global
  wires:
  current_sequence_avg/3(i_grid_neg_xi_avg) -> [i_grid_neg_xi_avg_mod2], sequences_current_control/3(i_neg_xi)
  grid_current_sampling_and_alpha_beta_transformation/1(i_grid_alpha) -> i_alphabeta2xieta/1(alpha)
  grid_current_sampling_and_alpha_beta_transformation/2(i_grid_beta) -> i_alphabeta2xieta/2(beta)
  [gamma_grid_pll_mod2] -> i_alphabeta2xieta/3(gamma)
  current_sequence_avg/2(i_grid_pos_eta_avg) -> sequences_current_control/2(i_pos_eta), [i_grid_pos_eta_avg_mod2]
  current_sequence_avg/1(i_grid_pos_xi_avg) -> sequences_current_control/1(i_pos_xi), [i_grid_pos_xi_avg_mod2]
  i_alphabeta2xieta/2(v_grid_pos_eta) -> current_sequence_avg/2(i_grid_pos_eta)
  ig_abc_pu/1 -> grid_current_sampling_and_alpha_beta_transformation/1(ig_abc)
  current_sequence_avg/4(i_grid_neg_eta_avg) -> [i_grid_neg_eta_avg_mod2], sequences_current_control/4(i_neg_eta)
  i_alphabeta2xieta/4(e) -> current_sequence_avg/4(i_grid_neg_eta)
  i_alphabeta2xieta/3(v_grid_neg_xi) -> current_sequence_avg/3(i_grid_neg_xi)
  i_alphabeta2xieta/1(xi) -> current_sequence_avg/1(i_grid_pos_xi)

== system afe_abc_inv_psm_n/afe_abc_inv_psm_mod2/AFE_control/afe_control/grid_voltage_phase_lock_loops ==
  ug_abc_pu : Inport
  DDSRF-PLL : Subsystem  Commented=on
  To Workspace1 : ToWorkspace  VariableName=gamma_grid_ddsrf_pll_sim_mod2  SampleTime=-1
      settings: MaxDataPoints=Ns_afe
  To Workspace2 : ToWorkspace  VariableName=omega_grid_ddsrf_pll_sim_mod2  SampleTime=-1
      settings: MaxDataPoints=Ns_afe
  To Workspace3 : ToWorkspace  VariableName=gamma_grid_dqpll_sim_mod2  SampleTime=-1
      settings: MaxDataPoints=Ns_afe
  To Workspace4 : ToWorkspace  VariableName=omega_grid_dqpll_sim_mod2  SampleTime=-1
      settings: MaxDataPoints=Ns_afe
  To Workspace5 : ToWorkspace  VariableName=gamma_grid_dqpll_ccaller_sim_mod2  SampleTime=-1
      settings: MaxDataPoints=Ns_afe
  To Workspace6 : ToWorkspace  VariableName=omega_grid_dqpll_ccaller_sim_mod2  SampleTime=-1
      settings: MaxDataPoints=Ns_afe
  Variant Source1 : VariantSource  VariantControls={use_advanced_pll == 1, use_dq_pll_ccaller_mod2 == 0, use_dq_pll_ccaller_mod2 == 1}
  Variant Source2 : VariantSource  VariantControls={use_advanced_pll == 1, use_dq_pll_ccaller_mod2 == 0, use_dq_pll_ccaller_mod2 == 1}
  dq_pll : Subsystem
  dq_pll_ccaller : Subsystem  Commented=on
  dqpll_ccaler mod2 : Scope  NumInputPorts=3
      settings: ActiveDisplayYMinimum=-0.88802937790751446  ActiveDisplayYMaximum=4.5431143753230572  DataLoggingVariableName=ScopeData4
  grid_plls_performance mod2 : Scope  NumInputPorts=3
      settings: ActiveDisplayYMinimum=-3.9265344417961696  ActiveDisplayYMaximum=3.9266424666979045
  tag scope: gamma_grid_pll_mod2=global, omega_grid_pll_mod2=global
  wires:
  [omega_grid_dqpll_ccaller] -> To Workspace6/1
  [gamma_grid_dqpll_ccaller] -> To Workspace5/1
  [omega_grid_dqpll] -> To Workspace4/1
  [gamma_grid_dqpll] -> To Workspace3/1
  [omega_grid_ddsrf_pll] -> To Workspace2/1
  [gamma_grid_ddsrf_pll] -> To Workspace1/1
  [omega_grid_pll_mod2] -> grid_plls_performance mod2/1  "omega_grid_pll_mod1"
  ug_abc_pu/1 -> dq_pll_ccaller/1(ug_abc_pu), DDSRF-PLL/1(ug_abc_pu), dq_pll/1(ug_abc_pu)
  dq_pll_ccaller/5(dqpll_state) -> dqpll_ccaler mod2/3  "dqpll_state"
  dq_pll_ccaller/4(dqpll_ueta) -> dqpll_ccaler mod2/2  "ueta_n"
  dq_pll_ccaller/3(dqpll_uxi) -> dqpll_ccaler mod2/1  "uxi_n"
  [gamma_grid_dqpll] -> grid_plls_performance mod2/2  "gamma_grid_dqpll"
  [gamma_grid_dqpll_ccaller] -> grid_plls_performance mod2/3  "gamma_grid_dqpll_ccaller"
  Variant Source2/1 -> [omega_grid_pll_mod2]
  [omega_grid_dqpll_ccaller] -> Variant Source2/3
  [omega_grid_dqpll] -> Variant Source2/2
  [omega_grid_ddsrf_pll] -> Variant Source2/1
  [gamma_grid_dqpll_ccaller] -> Variant Source1/3
  [gamma_grid_dqpll] -> Variant Source1/2
  [gamma_grid_ddsrf_pll] -> Variant Source1/1
  dq_pll_ccaller/2(omega_pu_hat) -> [omega_grid_dqpll_ccaller]
  dq_pll_ccaller/1(gamma_hat) -> [gamma_grid_dqpll_ccaller]
  dq_pll/1(gamma_grid_dqpll) -> [gamma_grid_dqpll]
  dq_pll/2(omega_grid_dqpll) -> [omega_grid_dqpll]
  DDSRF-PLL/2(omega_grid_ddsrf_pll) -> [omega_grid_ddsrf_pll]
  DDSRF-PLL/1(gamma_grid_ddsrf_pll) -> [gamma_grid_ddsrf_pll]
  Variant Source1/1 -> [gamma_grid_pll_mod2]

== system afe_abc_inv_psm_n/afe_abc_inv_psm_mod2/AFE_control/afe_control/grid_voltage_sequences ==
  grid_voltage_sampling_and_alpha_beta_transformation : Subsystem
  v_alphabeta2xieta : Subsystem
  voltage_sequence_avg : Subsystem
  tag scope: ug_alpha_pu_mod2=global, ug_beta_pu_mod2=global, v_grid_neg_eta_avg_mod2=global, v_grid_neg_xi_avg_mod2=global, v_grid_pos_eta_avg_mod2=global, v_grid_pos_xi_avg_mod2=global
  wires:
  [ugd_abc_pu_mod2] -> grid_voltage_sampling_and_alpha_beta_transformation/1(v_abc)
  grid_voltage_sampling_and_alpha_beta_transformation/1(u_grid_alpha) -> v_alphabeta2xieta/1(alpha), [ug_alpha_pu_mod2]
  v_alphabeta2xieta/1(xi) -> voltage_sequence_avg/1(v_grid_pos_xi)  "pos_xi"
  voltage_sequence_avg/1(v_grid_pos_xi_avg) -> [v_grid_pos_xi_avg_mod2]
  grid_voltage_sampling_and_alpha_beta_transformation/2(u_grid_beta) -> v_alphabeta2xieta/2(beta), [ug_beta_pu_mod2]
  voltage_sequence_avg/4(v_grid_neg_eta_avg) -> [v_grid_neg_eta_avg_mod2]
  voltage_sequence_avg/2(v_grid_pos_eta_avg) -> [v_grid_pos_eta_avg_mod2]
  voltage_sequence_avg/3(v_grid_neg_xi_avg) -> [v_grid_neg_xi_avg_mod2]
  v_alphabeta2xieta/3(v_grid_neg_xi) -> voltage_sequence_avg/3(v_grid_neg_xi)  "neg_xi"
  [gamma_grid_pll_mod2] -> v_alphabeta2xieta/3(gamma)
  v_alphabeta2xieta/2(eta) -> voltage_sequence_avg/2(v_grid_pos_eta)  "pos_eta"
  v_alphabeta2xieta/4(v_grid_neg_eta) -> voltage_sequence_avg/4(v_grid_neg_eta)  "neg_eta"

== system afe_abc_inv_psm_n/afe_abc_inv_psm_mod2/AFE_control/afe_control/ig afe quantizzation and one step delay ==
  ig_abc_pu : Inport
  Demux1 : Demux  Outputs=3
  Mux1 : Mux  Inputs=3
  ig afe quantizzation and one step delay : Subsystem
  igd_abc_pu : Outport
  wires:
  ig afe quantizzation and one step delay/3(igd_w_pu) -> Mux1/3
  ig afe quantizzation and one step delay/1(igd_u_pu) -> Mux1/1
  ig afe quantizzation and one step delay/2(igd_v_pu) -> Mux1/2
  Demux1/3 -> ig afe quantizzation and one step delay/3(ig_w_pu)
  Mux1/1 -> igd_abc_pu/1
  ig_abc_pu/1 -> Demux1/1
  Demux1/2 -> ig afe quantizzation and one step delay/2(ig_v_pu)
  Demux1/1 -> ig afe quantizzation and one step delay/1(ig_u_pu)

== system afe_abc_inv_psm_n/afe_abc_inv_psm_mod2/AFE_control/afe_control/instantaneus_power ==
  Demux2 : Demux  Outputs=3
  Demux3 : Demux  Outputs=3
  Gain : Gain  Gain=Vgrid_phase_normalization_factor
  Gain1 : Gain  Gain=Vgrid_phase_normalization_factor
  Gain2 : Gain  Gain=3/2
  Gain3 : Gain  Gain=3/2
  Gain4 : Gain  Gain=Vgrid_phase_normalization_factor
  Gain5 : Gain  Gain=Igrid_phase_normalization_factor
  Gain6 : Gain  Gain=Igrid_phase_normalization_factor
  Gain7 : Gain  Gain=Igrid_phase_normalization_factor
  Gain8 : Gain  Gain=1e-3
  Gain9 : Gain  Gain=1e-3
  Product{,1..3} (4 alike) : Product  RndMeth=Zero
  Sum : Sum  Inputs=|++
  Sum1 : Sum  Inputs=|+-
  To Workspace1 : ToWorkspace  VariableName=ug_b_rms__mod2_sim  SampleTime=-1
      settings: MaxDataPoints=Ns_afe
  To Workspace2 : ToWorkspace  VariableName=ug_a_rms__mod2_sim  SampleTime=-1
      settings: MaxDataPoints=Ns_afe
  To Workspace3 : ToWorkspace  VariableName=ug_c_rms__mod2_sim  SampleTime=-1
      settings: MaxDataPoints=Ns_afe
  To Workspace4 : ToWorkspace  VariableName=ig_b_rms__mod2_sim  SampleTime=-1
      settings: MaxDataPoints=Ns_afe
  To Workspace5 : ToWorkspace  VariableName=ig_a_rms__mod2_sim  SampleTime=-1
      settings: MaxDataPoints=Ns_afe
  To Workspace6 : ToWorkspace  VariableName=ig_c_rms__mod2_sim  SampleTime=-1
      settings: MaxDataPoints=Ns_afe
  To Workspace7 : ToWorkspace  VariableName=pwr_act_grid_mod2_sim  SampleTime=-1
      settings: MaxDataPoints=Ns_afe
  To Workspace8 : ToWorkspace  VariableName=pwr_react_grid_mod2_sim  SampleTime=-1
      settings: MaxDataPoints=Ns_afe
  abc2alphabeta : Subsystem
  "abc2alphabeta " : Subsystem
  moving_avarage_p : Subsystem
  moving_avarage_q : Subsystem
  rms : Subsystem
  rms1 : Subsystem
  rms2 : Subsystem
  rms3 : Subsystem
  rms4 : Subsystem
  rms5 : Subsystem
  tag scope: pwr_act_grid_mod2=global, pwr_react_grid_mod2=global
  wires:
  [igd_abc_pu_mod2] -> Demux3/1
  [ugd_abc_pu_mod2] -> Demux2/1
  Gain9/1 -> [pwr_react_grid_mod2]
  Gain8/1 -> [pwr_act_grid_mod2]
  Gain7/1 -> "abc2alphabeta "/3(c), rms5/1(In1)
  Gain6/1 -> "abc2alphabeta "/2(b), rms4/1(In1)
  Gain5/1 -> "abc2alphabeta "/1(a), rms3/1(In1)
  Gain4/1 -> abc2alphabeta/3(c), rms2/1(In1)
  Gain1/1 -> abc2alphabeta/2(b), rms1/1(In1)
  Gain/1 -> abc2alphabeta/1(a), rms/1(In1)
  Demux3/3 -> Gain7/1
  Demux3/2 -> Gain6/1
  Demux3/1 -> Gain5/1
  Demux2/3 -> Gain4/1
  Demux2/2 -> Gain1/1
  Demux2/1 -> Gain/1
  moving_avarage_q/1(out) -> Gain9/1
  moving_avarage_p/1(out) -> Gain8/1
  rms3/1(Out1) -> To Workspace5/1
  rms4/1(Out1) -> To Workspace4/1
  rms5/1(Out1) -> To Workspace6/1
  rms1/1(Out1) -> To Workspace1/1
  rms2/1(Out1) -> To Workspace3/1
  rms/1(Out1) -> To Workspace2/1
  Gain3/1 -> moving_avarage_q/1(in), To Workspace8/1
  Gain2/1 -> To Workspace7/1, moving_avarage_p/1(in)
  Sum/1 -> Gain2/1
  Sum1/1 -> Gain3/1
  Product3/1 -> Sum1/2
  Product2/1 -> Sum1/1
  Product1/1 -> Sum/2
  Product/1 -> Sum/1
  "abc2alphabeta "/1("alpha ") -> Product/2, Product2/2
  abc2alphabeta/1("alpha ") -> Product/1, Product3/2
  "abc2alphabeta "/2("beta ") -> Product3/1, Product1/2
  abc2alphabeta/2("beta ") -> Product2/1, Product1/1

== system afe_abc_inv_psm_n/afe_abc_inv_psm_mod2/AFE_control/afe_control/interesting scopes ==
  current_sequences_mod2 : Scope  NumInputPorts=4
      settings: ActiveDisplayYMinimum=-0.90637830615781712  ActiveDisplayYMaximum=0.328201162362058  DataLoggingVariableName=ScopeData2
  i_grid_seq_ref : Scope
      settings: ActiveDisplayYMinimum=-1.125  ActiveDisplayYMaximum=0.125
  voltage_sequences_mod2 : Scope  NumInputPorts=4
      settings: ActiveDisplayYMinimum=-0.11648824178726357  ActiveDisplayYMaximum=1.0452153910257462
  wires:
  [i_grid_seq_ref_mod2] -> i_grid_seq_ref/1  "i_grid_seq_ref"
  [i_grid_pos_eta_avg_mod2] -> current_sequences_mod2/2  "i_grid_pos_eta"
  [v_grid_pos_xi_avg_mod2] -> voltage_sequences_mod2/1  "u_grid_pos_xi"
  [i_grid_neg_eta_avg_mod2] -> current_sequences_mod2/4  "i_grid_neg_eta"
  [i_grid_pos_xi_avg_mod2] -> current_sequences_mod2/1  "i_grid_pos_xi"
  [v_grid_neg_xi_avg_mod2] -> voltage_sequences_mod2/3  "u_grid_neg_xi"
  [v_grid_pos_eta_avg_mod2] -> voltage_sequences_mod2/2  "u_grid_pos_eta"
  [i_grid_neg_xi_avg_mod2] -> current_sequences_mod2/3  "i_grid_neg_xi"
  [v_grid_neg_eta_avg_mod2] -> voltage_sequences_mod2/4  "u_grid_neg_eta"

== system afe_abc_inv_psm_n/afe_abc_inv_psm_mod2/AFE_control/afe_control/is afe quantizzation and one step delay ==
  is_abc_pu : Inport
  Demux : Demux  Outputs=3
  Mux : Mux  Inputs=3
  is afe quantizzation and one step delay : Subsystem
  isd_abc_pu : Outport
  wires:
  Demux/2 -> is afe quantizzation and one step delay/2(is_v_pu)
  Demux/3 -> is afe quantizzation and one step delay/3(is_w_pu)
  Mux/1 -> isd_abc_pu/1
  Demux/1 -> is afe quantizzation and one step delay/1(is_u_pu)
  is afe quantizzation and one step delay/1(isd_u_pu) -> Mux/1
  is afe quantizzation and one step delay/3(isd_w_pu) -> Mux/3
  is_abc_pu/1 -> Demux/1
  is afe quantizzation and one step delay/2(isd_v_pu) -> Mux/2

== system afe_abc_inv_psm_n/afe_abc_inv_psm_mod2/AFE_control/afe_control/islanding_mode_detector ==
  gamma : Inport
  alpha : Inport  Port=2
  beta : Inport  Port=3
  Gain : Gain  Gain=7
  MATLAB Function : MATLAB Function  TreatAsAtomicUnit=on
  To Workspace20 : ToWorkspace  VariableName=u_7th_eta_sim_mod2  SampleTime=-1
      settings: MaxDataPoints=Ns_afe
  To Workspace21 : ToWorkspace  VariableName=u_7th_xi_sim_mod2  SampleTime=-1
      settings: MaxDataPoints=Ns_afe
  bounder : MATLAB Function  TreatAsAtomicUnit=on
  moving_avarage_1 : Subsystem
  moving_avarage_2 : Subsystem
  seventh_ugrid_component mod2 : Scope  NumInputPorts=2
      settings: ActiveDisplayYMinimum=-0.19805169308492759  ActiveDisplayYMaximum=0.20219237067929344  DataLoggingVariableName=ScopeData10
  tag scope: u_7th_eta_avg_mod2=global, u_7th_xi_avg_mod2=global
  wires:
  moving_avarage_2/1(y) -> seventh_ugrid_component mod2/2, [u_7th_eta_avg_mod2]  "u_7th_eta"
  moving_avarage_1/1(y) -> seventh_ugrid_component mod2/1, [u_7th_xi_avg_mod2]  "u_7th_xi"
  [u_7th_eta_avg_mod2] -> To Workspace20/1
  [u_7th_xi_avg_mod2] -> To Workspace21/1
  MATLAB Function/2(eta) -> moving_avarage_2/1(u)
  beta/1 -> MATLAB Function/2(beta)  "u_grid_beta"
  alpha/1 -> MATLAB Function/1(alpha)  "u_grid_alpha"
  Gain/1 -> bounder/1(u)
  bounder/1(y) -> MATLAB Function/3(gamma)
  MATLAB Function/1(xi) -> moving_avarage_1/1(u)
  gamma/1 -> Gain/1  "gamma_grid"

== system afe_abc_inv_psm_n/afe_abc_inv_psm_mod2/AFE_control/afe_control/phase_compensation_1 ==
  local_time : Inport
  master_time : Inport  Port=2
  alignment_ctrl : Subsystem
  y : Outport
  wires:
  local_time/1 -> alignment_ctrl/1(local_time)
  master_time/1 -> alignment_ctrl/2(master_time)
  alignment_ctrl/1(dp) -> y/1
